simulink model "MotionControl"  (R2024b)
settings: Solver=VariableStepAuto  StartTime=0.0  StopTime=10.0  RelTol=1e-3
model workspace (MAT data in the model file):
  DesLinVel = Simulink.Parameter
  DesLinVel.Value = 0.3
  DesLinVel.Complexity = 'real'
  DesLinVel.Dimensions = [1 1]
  DesLinVel.DataType = 'auto'
  LookaheadDist = Simulink.Parameter
  LookaheadDist.Value = 2
  LookaheadDist.Complexity = 'real'
  LookaheadDist.Dimensions = [1 1]
  LookaheadDist.DataType = 'auto'
undefined symbols (not defined in the file): waypoints
libraries: robotalgslib x1
settings Model: DataDictionary=DataDictionary.sldd  ParameterArgumentNames=DesLinVel,LookaheadDist  Creator=charber  LastModifiedBy=tsamak

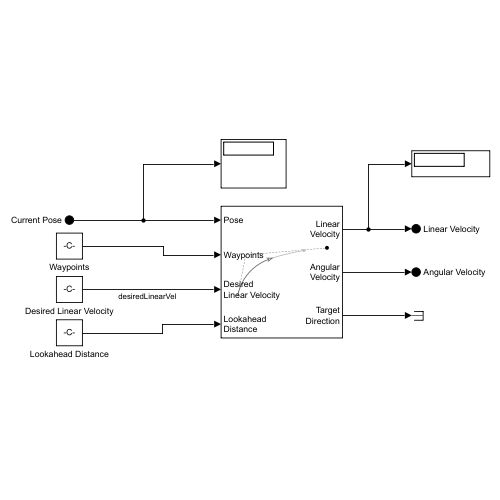
[thumbnail: Simulink's stored preview of the top-level diagram]
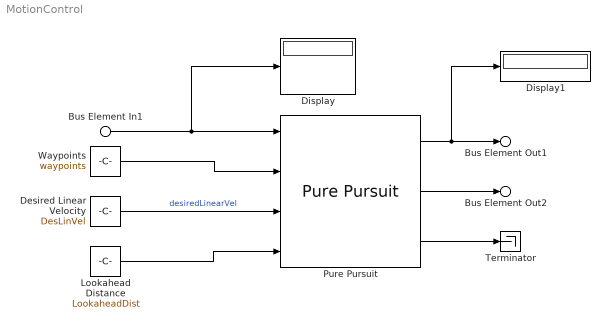
== system MotionControl ==
  Bus Element In1 : Inport  PortName=Current Pose
  Desired Linear Velocity : Constant  Value=DesLinVel
  Display : Display
  Display1 : Display
  Lookahead Distance : Constant  Value=LookaheadDist
  Pure Pursuit : robotalgslib/Pure Pursuit  DesiredLinearVelocityPort=on  DesiredLinearVelocity=0.3  MaxAngularVelocity=1.0  LookaheadDistancePort=on  LookaheadDistance=2.0  TargetDirPort=on  SimulateUsing=Code generation
  Terminator : Terminator
  Waypoints : Constant  Value=waypoints
  Bus Element Out1 : Outport  PortName=Linear Velocity
  Bus Element Out2 : Outport  Port=2  PortName=Angular Velocity
  wires:
  Lookahead Distance/1 -> Pure Pursuit/4
  Pure Pursuit/1 -> Display1/1, Bus Element Out1/1
  Pure Pursuit/2 -> Bus Element Out2/1
  Pure Pursuit/3 -> Terminator/1
  Waypoints/1 -> Pure Pursuit/2
  Desired Linear Velocity/1 -> Pure Pursuit/3  "desiredLinearVel"
  Bus Element In1/1 -> Display/1, Pure Pursuit/1
